simulink subsystem "DataAssimilationInterface"  (R2025a)
settings: Solver=VariableStepAuto  StartTime=0.0  StopTime=10.0  RelTol=1e-3
settings Model: Creator=yvijay  LastModifiedBy=atcushen

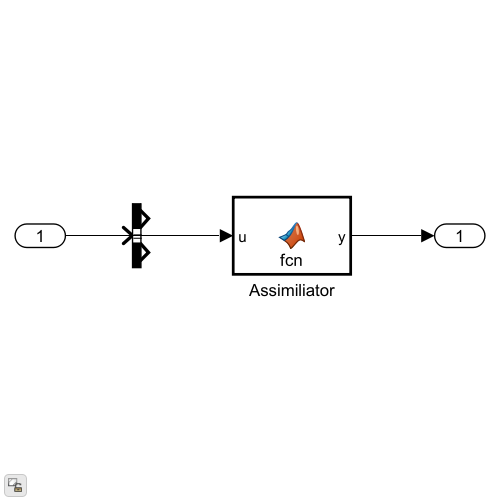
[thumbnail: Simulink's stored preview of the top-level diagram]
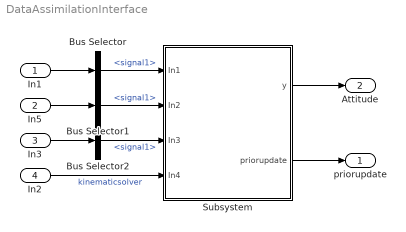
== system DataAssimilationInterface ==
  In1 : Inport
  In5 : Inport  Port=2
  In3 : Inport  Port=3
  In2 : Inport  Port=4
  Bus Selector : BusSelector  OutputSignals=signal1
  Bus Selector1 : BusSelector  OutputSignals=signal1
  Bus Selector2 : BusSelector  OutputSignals=signal1
  Subsystem : Subsystem
  priorupdate : Outport
  Attitude : Outport  Port=2
  wires:
  In1/1 -> Bus Selector/1
  Subsystem/2(priorupdate) -> priorupdate/1
  Subsystem/1(y) -> Attitude/1
  In3/1 -> Bus Selector2/1
  Bus Selector/1 -> Subsystem/1(In1)  "<signal1>"
  Bus Selector1/1 -> Subsystem/2(In2)  "<signal1>"
  Bus Selector2/1 -> Subsystem/3(In3)  "<signal1>"
  In2/1 -> Subsystem/4(In4)  "kinematicsolver"
  In5/1 -> Bus Selector1/1

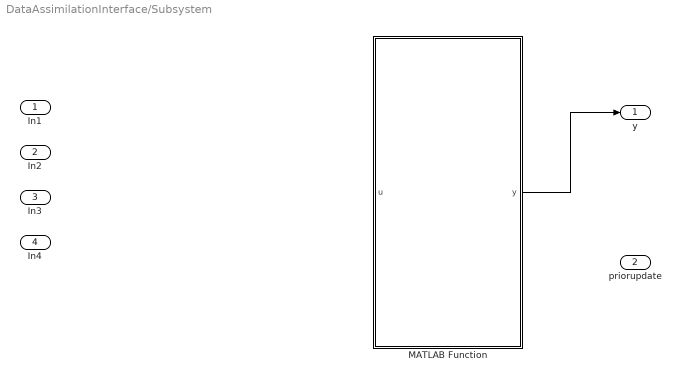
== system DataAssimilationInterface/Subsystem ==
  In1 : Inport
  In2 : Inport  Port=2
  In3 : Inport  Port=3
  In4 : Inport  Port=4
  MATLAB Function : MATLAB Function  TreatAsAtomicUnit=on
  y : Outport
  priorupdate : Outport  Port=2
  wires:
  ? -> priorupdate/1
  MATLAB Function/1(y) -> y/1

== matlab function DataAssimilationInterface/Subsystem/MATLAB Function ==
  data: u input; y output
function y  = fcn(u)

y = u;
